simulink model "cluster_control_1_dx"  (R2016a)
settings: Solver=VariableStepAuto  StartTime=0.0  StopTime=10.0  RelTol=1e-3
undefined symbols (not defined in the file): L1, x0
settings Model: Creator=richa  LastModifiedBy=richa

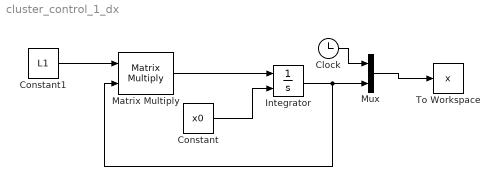
== system cluster_control_1_dx ==
  Clock : Clock
  Constant : Constant  Value=x0
  Constant1 : Constant  Value=L1  VectorParams1D=off
  Integrator : Integrator  InitialConditionSource=external
  Matrix Multiply : Product  Multiplication=Matrix(*)
  Mux : Mux  Inputs=2
  To Workspace : ToWorkspace  VariableName=x  SampleTime=-1
  wires:
  Constant/1 -> Integrator/2
  Mux/1 -> To Workspace/1
  Clock/1 -> Mux/1
  Matrix Multiply/1 -> Integrator/1
  Constant1/1 -> Matrix Multiply/1
  Integrator/1 -> Mux/2, Matrix Multiply/2
